simulink model "test_ml_neuron_v2"  (R2018a)
settings: Solver=VariableStepAuto  StartTime=0.0  StopTime=1  MaxStep=1e-4  RelTol=1e-3
libraries: fl_lib x8, nesl_utility x2
settings Model: Creator=bici  LastModifiedBy=bici
settings DataIOCC: SaveState=on  InspectSignalLogs=on

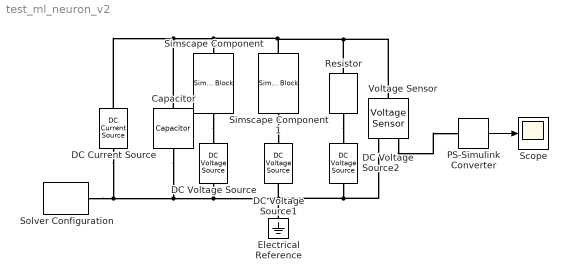
== system test_ml_neuron_v2 ==
  Capacitor : fl_lib/Electrical/Electrical Elements/Capacitor  c=20 uF  r=0 Ohm  g=0 1/Ohm  i_specify=off  i_priority=None  i=0 A  i_nominal_specify=off  i_nominal_unit=A  i_nominal_value=1  v_specify=off  v_priority=None  v=-10 mV  v_nominal_specify=off  v_nominal_unit=V  v_nominal_value=1  vc_specify=on  vc_priority=High  vc=-10 mV  vc_nominal_specify=off  vc_nominal_unit=V  vc_nominal_value=1
  DC Current Source : fl_lib/Electrical/Electrical Sources/DC Current Source  i0=85 uA
      settings: SourceProductName=Simscape  SourceProductBaseCode=SS
  DC Voltage Source : fl_lib/Electrical/Electrical Sources/DC Voltage Source  v0=120 mV
  DC Voltage Source1 : fl_lib/Electrical/Electrical Sources/DC Voltage Source  v0=-84 mV
  DC Voltage Source2 : fl_lib/Electrical/Electrical Sources/DC Voltage Source  v0=-60 mV
  Electrical Reference : fl_lib/Electrical/Electrical Elements/Electrical Reference
  PS-Simulink Converter : nesl_utility/PS-Simulink Converter  PhysicalDomain=network_engine_domain  SubClassName=ps_output  LeftPortType=input  RightPortType=output  PseudoPeriodic=off  Frequencies=[]  Unit=1  AffineConversion=off
  Resistor : fl_lib/Electrical/Electrical Elements/Resistor  R=1/0.002 Ohm  i_specify=off  i_priority=None  i=0 A  i_nominal_specify=off  i_nominal_unit=A  i_nominal_value=1  v_specify=off  v_priority=None  v=40 mV  v_nominal_specify=off  v_nominal_unit=V  v_nominal_value=1
  Scope : Scope
  Simscape Component : SimscapeComponentBlock  SourceFile=resistor_morris_lecar  ComponentPath=resistor_morris_lecar  ComponentVariants=resistor_morris_lecar  ComponentVariantNames=resistor_morris_lecar  ClassName=resistor_morris_lecar  SchemaVersion=1  g=4.4 mS  V1=-1.2 mV  V2=18 mV  E=120 mV  M_inf_specify=off  M_inf_priority=None  M_inf=5e-4  M_inf_nominal_specify=off  M_inf_nominal_unit=1  M_inf_nominal_value=1  i_specify=off  i_priority=None  i=0 A  i_nominal_specify=off  i_nominal_unit=A  i_nominal_value=1  v_specify=off  v_priority=None  v=0 V  v_nominal_specify=off  v_nominal_unit=V  v_nominal_value=1  memductance_specify=off  memductance_priority=None  memductance=0 mS  memductance_nominal_specify=off  memductance_nominal_unit=mS  memductance_nominal_value=1
      settings: CopyFcn=simscape.engine.sli.internal.componentblockcallback(gcbh,'COPY')  PreCopyFcn=simscape.engine.sli.internal.componentblockcallback(gcbh,'PRECOPY')  PreDeleteFcn=simscape.engine.sli.internal.componentblockcallback(gcbh,'PREDELETE')
      mask Type: resistor_morris_lecar
      mask Display:
      | disp('Simscape\n\n\n')
      | disp('\n\n\nresistor_morris_lecar');
      | color('red');
      | port_label('RConn', 1,'-');
      | port_label('LConn', 1,'+');
  Simscape Component1 : SimscapeComponentBlock  SourceFile=memristor_morris_lecar  ComponentPath=memristor_morris_lecar  ComponentVariants=memristor_morris_lecar  ComponentVariantNames=memristor_morris_lecar  ClassName=memristor_morris_lecar  SchemaVersion=1  g=8 mS  V3=2 mV  V4=30 mV  lambda_N=0.04 1/ms  E=-84 mV  N_specify=off  N_priority=None  N=0  N_nominal_specify=off  N_nominal_unit=1  N_nominal_value=1  N_inf_specify=off  N_inf_priority=None  N_inf=5e-4  N_inf_nominal_specify=off  N_inf_nominal_unit=1  N_inf_nominal_value=1  lambda_specify=off  lambda_priority=None  lambda=0 1/ms  lambda_nominal_specify=off  lambda_nominal_unit=1/ms  lambda_nominal_value=1  i_specify=off  i_priority=None  i=0 A  i_nominal_specify=off  i_nominal_unit=A  i_nominal_value=1  v_specify=off  v_priority=None  v=0 V  v_nominal_specify=off  v_nominal_unit=V  v_nominal_value=1  memductance_specify=off  memductance_priority=None  memductance=0 mS  memductance_nominal_specify=off  memductance_nominal_unit=mS  memductance_nominal_value=1
      settings: CopyFcn=simscape.engine.sli.internal.componentblockcallback(gcbh,'COPY')  PreCopyFcn=simscape.engine.sli.internal.componentblockcallback(gcbh,'PRECOPY')  PreDeleteFcn=simscape.engine.sli.internal.componentblockcallback(gcbh,'PREDELETE')
      mask Type: memristor_morris_lecar
      mask Display:
      | disp('Simscape\n\n\n')
      | disp('\n\n\nmemristor_morris_lecar');
      | color('red');
      | port_label('RConn', 1,'-');
      | port_label('LConn', 1,'+');
  Solver Configuration : nesl_utility/Solver Configuration  PhysicalDomain=network_engine_domain  SubClassName=solver  LeftPortType=input  RightPortType=generic  Tones=[]  Harmonics=[]  SimulateNoise=off  Profile=off  UseLocalSampling=off  EnableSwitchedLinearOptims=on  FrequencyDomain=off  UseCCode=off  RelTol=0.001  AbsTol=1e-06  MinStep=1e-09  ToWorkspace=off  RevertToSquareIcSolve=off  NumHomotopyIterations=100  PhasorMode=off  PhasorModeNumHarmonics=1  DoDC=off  ResidualTolerance=1e-09  UseLocalSolver=off  LocalSolverChoice=NE_BACKWARD_EULER_ADVANCER  LocalSolverSampleTime=0.001  DoFixedCost=off  MaxNonlinIter=3  MaxModeIter=2  LinearAlgebra=Sparse  EquationFormulation=NE_TIME_EF  DelaysMemoryBudget=1024  AutomaticFiltering=on  FilteringTimeConstant=0.001
  Voltage Sensor : fl_lib/Electrical/Electrical Sensors/Voltage Sensor
  wires:
  PS-Simulink Converter/1 -> Scope/1
  connections:
  Electrical Reference/LConn1 -- Voltage Sensor/RConn2 -- DC Voltage Source2/RConn1 -- DC Current Source/RConn1 -- Solver Configuration/RConn1 -- Capacitor/RConn1 -- DC Voltage Source/RConn1 -- DC Voltage Source1/RConn1
  Resistor/RConn1 -- DC Voltage Source2/LConn1
  Simscape Component/RConn1 -- DC Voltage Source/LConn1
  Simscape Component1/RConn1 -- DC Voltage Source1/LConn1
  Capacitor/LConn1 -- DC Current Source/LConn1 -- Voltage Sensor/LConn1 -- Resistor/LConn1 -- Simscape Component1/LConn1 -- Simscape Component/LConn1
  Voltage Sensor/RConn1 -- PS-Simulink Converter/LConn1
